simulink model "Lab1_6F"  (R2018a)
settings: Solver=VariableStepAuto  StartTime=0.0  StopTime=180  RelTol=1e-3
settings Model: Creator=melab2  LastModifiedBy=rahul

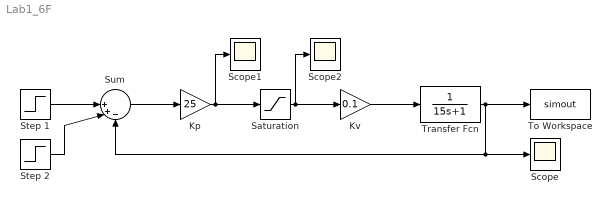
== system Lab1_6F ==
  Kp : Gain  Gain=25
  Kv : Gain  Gain=0.1
  Saturation : Saturate  UpperLimit=25  LowerLimit=-75
  Scope : Scope
  Scope1 : Scope
  Scope2 : Scope
  "Step 1 " : Step  SampleTime=0
  Step 2 : Step  Time=75  After=-2  SampleTime=0
  Sum : Sum  Inputs=||++-
  To Workspace : ToWorkspace  VariableName=simout  SampleTime=-1
  Transfer Fcn : TransferFcn  Denominator=[15 1]
  wires:
  Sum/1 -> Kp/1
  Kv/1 -> Transfer Fcn/1
  Transfer Fcn/1 -> Sum/3, Scope/1, To Workspace/1
  "Step 1 "/1 -> Sum/1
  Step 2/1 -> Sum/2
  Kp/1 -> Scope1/1, Saturation/1
  Saturation/1 -> Scope2/1, Kv/1
